simulink model "model3"  (R2023a)
settings: Solver=ode4  StartTime=0.0  StopTime=1000  FixedStep=simulation_dt  RelTol=1e-3
undefined symbols (not defined in the file or in its folder): input, k_harmonics, magnitude, simulation_dt
libraries: simulink x2
settings Model: Creator=dionl  LastModifiedBy=dionl

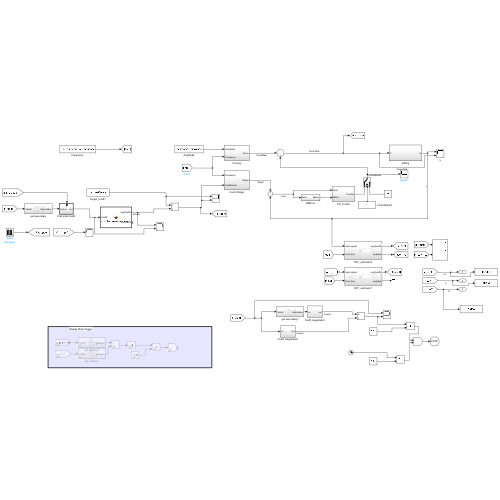
[thumbnail: Simulink's stored preview of the top-level diagram]
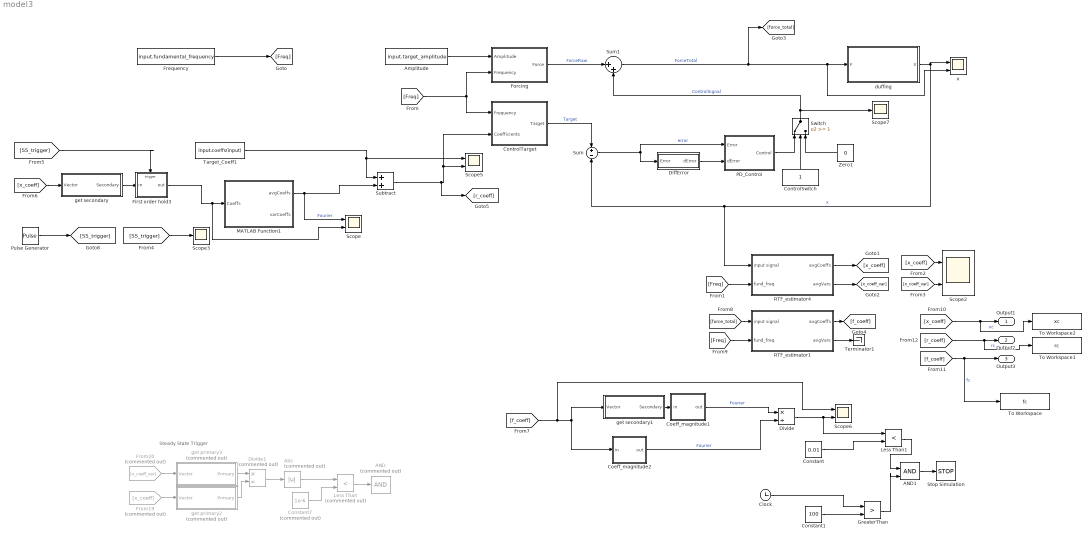
== system model3 ==
  note: Steady State Trigger
  AND : Logic  Commented=on  Inputs=1  IconShape=distinctive  AllPortsSameDT=off  OutDataTypeStr=boolean
  AND1 : Logic  IconShape=distinctive  AllPortsSameDT=off  OutDataTypeStr=boolean
  Abs : Abs  Commented=on  SaturateOnIntegerOverflow=off
  Amplitude : Constant  Value=input.target_amplitude
  Clock : Clock
  Coeff_magnitude1 : Subsystem
  Coeff_magnitude2 : Subsystem
  Constant : Constant  Value=0.01
  Constant1 : Constant  Value=100
  Constant7 : Constant  Commented=on  Value=1e-6
  ControlSwitch : Constant
  ControlTarget : Subsystem
  DiffError : Subsystem
  Divide : Product  Inputs=*/
  Divide1 : Product  Commented=on  Inputs=*/
  First order hold3 : Subsystem  TreatAsAtomicUnit=on
  Forcing : Subsystem
  Frequency : Constant  Value=input.fundamental_frequency
  From19 : From  Commented=on  GotoTag=x_coeff
  From20 : From  Commented=on  GotoTag=x_coeff_var
  GreaterThan : RelationalOperator  Operator=>  OutDataTypeStr=boolean  RndMeth=Simplest  InputSameDT=off
  Less Than : RelationalOperator  Commented=on  Operator=<  OutDataTypeStr=boolean  RndMeth=Simplest  InputSameDT=off
  Less Than1 : RelationalOperator  Operator=<  OutDataTypeStr=boolean  RndMeth=Simplest  InputSameDT=off
  MATLAB Function1 : MATLAB Function  TreatAsAtomicUnit=on
  PD_Control : Subsystem
  Pulse Generator : DiscretePulseGenerator  PulseType=Time based  Period=50  PulseWidth=5  PhaseDelay=simulation_dt
  RTF_estimator1 : Subsystem
  RTF_estimator4 : Subsystem
  Scope{,2,5..6} (4 alike) : Scope  NumInputPorts=2
  Scope3 : Scope
  Scope7 : Scope
  Stop Simulation : Stop
  Subtract : Sum
  Sum : Sum  Inputs=+|-
  Sum1 : Sum  Inputs=|++
  Switch : Switch  Threshold=1  SaturateOnIntegerOverflow=off  InputSameDT=off
  Target_Coeff1 : Constant  Value=input.coeffs(input)
  Terminator1 : Terminator
  To Workspace : ToWorkspace  VariableName=fc  SaveFormat=Timeseries  SampleTime=-1
  To Workspace1 : ToWorkspace  VariableName=rc  SaveFormat=Timeseries  SampleTime=-1
  To Workspace2 : ToWorkspace  VariableName=xc  SaveFormat=Timeseries  SampleTime=-1
  Zero1 : Constant  Value=0
  duffing : Subsystem
  get primary2 : Subsystem  Commented=on
  get primary3 : Subsystem  Commented=on
  get secondary : Subsystem
  get secondary1 : Subsystem
  x : Scope  NumInputPorts=2
  Output1 : Outport
  Output2 : Outport  Port=2
  Output3 : Outport  Port=3
  wires:
  Subtract/1 -> [r_coeff], Scope5/2, ControlTarget/2(Coefficients)
  Switch/1 -> Sum1/2, Scope7/1  "ControlSignal"
  Zero1/1 -> Switch/3
  Sum1/1 -> [force_total], x/2, duffing/1(F)  "ForceTotal"
  PD_Control/1(Control) -> Switch/1
  duffing/1(X) -> x/1, RTF_estimator4/1(input signal), Sum/2  "x"
  DiffError/1(dError) -> PD_Control/2(dError)
  Forcing/1(Force) -> Sum1/1  "ForceRaw"
  ControlSwitch/1 -> Switch/2
  Amplitude/1 -> Forcing/1(Amplitude)
  ControlTarget/1(Target) -> Sum/1  "Target"
  Frequency/1 -> [Freq]
  Sum/1 -> PD_Control/1(Error), DiffError/1(Error)  "error"
  [Freq] -> ControlTarget/1(Frequency), Forcing/2(Frequency)
  [Freq] -> RTF_estimator4/2(fund_freq)
  get primary3/1(Primary) -> Divide1/1
  Less Than/1 -> AND/1
  get primary2/1(Primary) -> Divide1/2
  Constant7/1 -> Less Than/2
  From20/1 -> get primary3/1(Vector)
  Divide1/1 -> Abs/1
  From19/1 -> get primary2/1(Vector)
  RTF_estimator4/2(avgVars) -> [x_coeff_var]
  RTF_estimator4/1(avgCoeffs) -> [x_coeff]
  [x_coeff_var] -> Scope2/2
  [x_coeff] -> Scope2/1
  [SS_trigger] -> Scope3/1
  Abs/1 -> Less Than/1
  Target_Coeff1/1 -> Subtract/1, Scope5/1
  [x_coeff] -> get secondary/1(Vector)
  get secondary/1(Secondary) -> First order hold3/1(in)
  get secondary1/1(Secondary) -> Coeff_magnitude1/1(in)
  Coeff_magnitude1/1(out) -> Divide/1  "Fourier"
  Coeff_magnitude2/1(out) -> Divide/2  "Fourier"
  Divide/1 -> Less Than1/1, Scope6/2
  [SS_trigger] -> First order hold3/Trigger
  Pulse Generator/1 -> [SS_trigger]
  [force_total] -> RTF_estimator1/1(input signal)
  [Freq] -> RTF_estimator1/2(fund_freq)
  RTF_estimator1/1(avgCoeffs) -> [f_coeff]
  RTF_estimator1/2(avgVars) -> Terminator1/1
  [f_coeff] -> Scope6/1, Coeff_magnitude2/1(in), get secondary1/1(Vector)
  Constant/1 -> Less Than1/2
  Less Than1/1 -> AND1/1
  [x_coeff] -> To Workspace2/1, Output1/1  "xc"
  [f_coeff] -> To Workspace/1, Output3/1  "fc"
  [r_coeff] -> To Workspace1/1, Output2/1  "rc"
  First order hold3/1(out) -> Scope/2, MATLAB Function1/1(Coeffs)
  MATLAB Function1/1(avgCoeffs) -> Scope/1, Subtract/2  "Fourier"
  Clock/1 -> GreaterThan/1
  Constant1/1 -> GreaterThan/2
  AND1/1 -> Stop Simulation/1
  GreaterThan/1 -> AND1/2

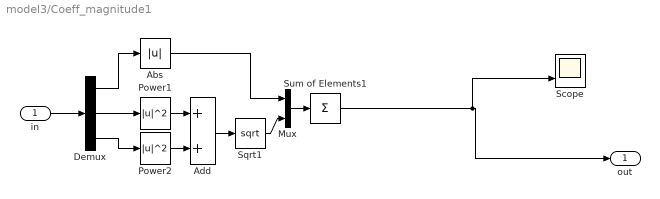
== system model3/Coeff_magnitude1 ==
  in : Inport
  Abs : Abs  SaturateOnIntegerOverflow=off
  Add : Sum
  Demux : Demux  Outputs=[1 k_harmonics k_harmonics]
  Mux : Mux  Inputs=2
  Power1 : Math  Operator=magnitude^2
  Power2 : Math  Operator=magnitude^2
  Scope : Scope  NumInputPorts=2
  Sqrt1 : Sqrt
  Sum of Elements1 : Sum  Inputs=+
  out : Outport
  wires:
  in/1 -> Demux/1
  Demux/1 -> Abs/1
  Demux/2 -> Power1/1
  Demux/3 -> Power2/1
  Power1/1 -> Add/1
  Power2/1 -> Add/2
  Add/1 -> Sqrt1/1
  Abs/1 -> Mux/1
  Sqrt1/1 -> Mux/2
  Mux/1 -> Sum of Elements1/1
  Sum of Elements1/1 -> Scope/2, out/1

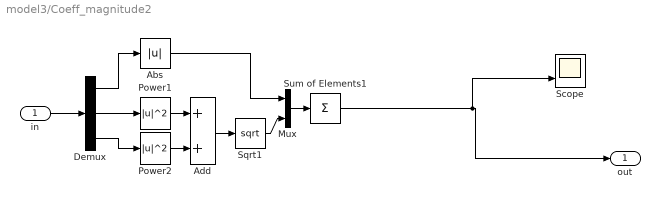
== system model3/Coeff_magnitude2 ==
  in : Inport
  Abs : Abs  SaturateOnIntegerOverflow=off
  Add : Sum
  Demux : Demux  Outputs=[1 k_harmonics k_harmonics]
  Mux : Mux  Inputs=2
  Power1 : Math  Operator=magnitude^2
  Power2 : Math  Operator=magnitude^2
  Scope : Scope  NumInputPorts=2
  Sqrt1 : Sqrt
  Sum of Elements1 : Sum  Inputs=+
  out : Outport
  wires:
  Sum of Elements1/1 -> out/1, Scope/2
  Mux/1 -> Sum of Elements1/1
  Sqrt1/1 -> Mux/2
  Abs/1 -> Mux/1
  Add/1 -> Sqrt1/1
  Power2/1 -> Add/2
  Power1/1 -> Add/1
  Demux/3 -> Power2/1
  Demux/2 -> Power1/1
  Demux/1 -> Abs/1
  in/1 -> Demux/1

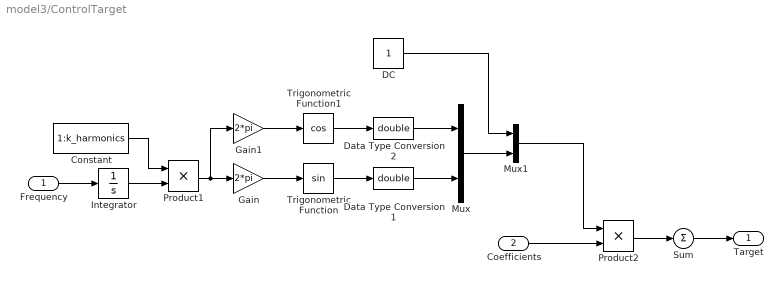
== system model3/ControlTarget ==
  Frequency : Inport
  Coefficients : Inport  Port=2
  Constant : Constant  Value=1:k_harmonics
  DC : Constant
  Data Type Conversion1 : DataTypeConversion  OutDataTypeStr=double  SaturateOnIntegerOverflow=off  RndMeth=Floor
  Data Type Conversion2 : DataTypeConversion  OutDataTypeStr=double  SaturateOnIntegerOverflow=off  RndMeth=Floor
  Gain : Gain  Gain=2*pi
  Gain1 : Gain  Gain=2*pi
  Integrator : Integrator
  Mux : Mux  Inputs=2
  Mux1 : Mux  Inputs=2
  Product1 : Product
  Product2 : Product  RndMeth=Zero
  Sum : Sum  Inputs=|+|
  Trigonometric Function : Trigonometry
  Trigonometric Function1 : Trigonometry  Operator=cos
  Target : Outport
  wires:
  Gain/1 -> Trigonometric Function/1
  Product2/1 -> Sum/1
  Gain1/1 -> Trigonometric Function1/1
  Sum/1 -> Target/1
  Frequency/1 -> Integrator/1
  Integrator/1 -> Product1/2
  Constant/1 -> Product1/1
  Trigonometric Function/1 -> Data Type Conversion1/1
  Mux1/1 -> Product2/1
  Trigonometric Function1/1 -> Data Type Conversion2/1
  Product1/1 -> Gain1/1, Gain/1
  Coefficients/1 -> Product2/2
  Data Type Conversion2/1 -> Mux/1
  Data Type Conversion1/1 -> Mux/2
  Mux/1 -> Mux1/2
  DC/1 -> Mux1/1

== system model3/DiffError ==
  Error : Inport
  Sum4 : Sum  Inputs=|-+
  Unit Delay : UnitDelay  SampleTime=-1  HasFrameUpgradeWarning=on
  Weighted Sample Time : SampleTimeMath  TsampMathOp=/
  dError : Outport
  wires:
  Unit Delay/1 -> Sum4/1
  Sum4/1 -> Weighted Sample Time/1
  Weighted Sample Time/1 -> dError/1
  Error/1 -> Unit Delay/1, Sum4/2

== system model3/First order hold3 ==
  in : Inport  LatchByDelayingOutsideSignal=on
  Trigger : TriggerPort  VariantControl=(inherit)
  out : Outport  InitialOutput=0
  wires:
  in/1 -> out/1

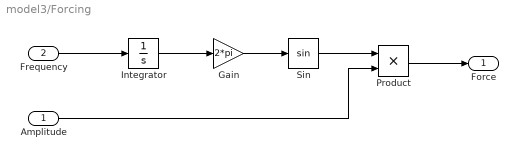
== system model3/Forcing ==
  Amplitude : Inport
  Frequency : Inport  Port=2
  Gain : Gain  Gain=2*pi
  Integrator : Integrator
  Product : Product
  Sin : Trigonometry
  Force : Outport
  wires:
  Frequency/1 -> Integrator/1
  Gain/1 -> Sin/1
  Amplitude/1 -> Product/2
  Integrator/1 -> Gain/1
  Sin/1 -> Product/1
  Product/1 -> Force/1

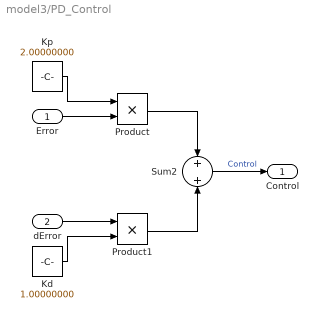
== system model3/PD_Control ==
  Error : Inport
  dError : Inport  Port=2
  Kd : Constant  Value=1.00000000
  Kp : Constant  Value=2.00000000
  Product : Product  RndMeth=Zero
  Product1 : Product  RndMeth=Zero
  Sum2 : Sum  Inputs=+|+
  Control : Outport
  wires:
  Kp/1 -> Product/1
  Kd/1 -> Product1/2
  Product/1 -> Sum2/1
  Product1/1 -> Sum2/2
  Error/1 -> Product/2
  Sum2/1 -> Control/1  "Control"
  dError/1 -> Product1/1

== system model3/RTF_estimator1 ==
  input signal : Inport
  fund_freq : Inport  Port=2
  MATLAB Function1 : MATLAB Function  TreatAsAtomicUnit=on
  Subsystem : Subsystem
  Terminator : Terminator
  avgCoeffs : Outport
  avgVars : Outport  Port=2
  wires:
  MATLAB Function1/1(avgCoeffs) -> avgCoeffs/1  "Fourier"
  MATLAB Function1/2(varCoeffs) -> avgVars/1
  Subsystem/1(Fourier1) -> MATLAB Function1/1(Coeffs)
  fund_freq/1 -> Subsystem/2(fund_freq)
  Subsystem/2(Phase1) -> Terminator/1
  input signal/1 -> Subsystem/1(input signal)

== system model3/RTF_estimator4 ==
  input signal : Inport
  fund_freq : Inport  Port=2
  MATLAB Function1 : MATLAB Function  TreatAsAtomicUnit=on
  Subsystem : Subsystem
  Terminator : Terminator
  avgCoeffs : Outport
  avgVars : Outport  Port=2
  wires:
  input signal/1 -> Subsystem/1(input signal)
  Subsystem/2(Phase1) -> Terminator/1
  fund_freq/1 -> Subsystem/2(fund_freq)
  Subsystem/1(Fourier1) -> MATLAB Function1/1(Coeffs)
  MATLAB Function1/2(varCoeffs) -> avgVars/1
  MATLAB Function1/1(avgCoeffs) -> avgCoeffs/1  "Fourier"

== system model3/duffing ==
  F : Inport
  Integrator : Integrator
  Integrator1 : Integrator
  MATLAB Function : MATLAB Function  TreatAsAtomicUnit=on
  X : Outport
  wires:
  Integrator1/1 -> MATLAB Function/2(v)
  MATLAB Function/2(dvdt) -> Integrator1/1
  MATLAB Function/1(dxdt) -> Integrator/1
  F/1 -> MATLAB Function/3(excitation)
  Integrator/1 -> MATLAB Function/1(x), X/1

== system model3/get primary2 ==
  Vector : Inport
  Demux : Demux  Outputs=[1, 1, k_harmonics-1, 1, k_harmonics-1]
  Mux : Mux  Inputs=2
  Terminator2 : Terminator
  Terminator3 : Terminator
  Terminator4 : Terminator
  Primary : Outport
  wires:
  Vector/1 -> Demux/1
  Demux/5 -> Terminator4/1
  Demux/3 -> Terminator3/1
  Mux/1 -> Primary/1
  Demux/4 -> Mux/2
  Demux/2 -> Mux/1
  Demux/1 -> Terminator2/1

== system model3/get primary3 ==
  Vector : Inport
  Demux : Demux  Outputs=[1, 1, k_harmonics-1, 1, k_harmonics-1]
  Mux : Mux  Inputs=2
  Terminator2 : Terminator
  Terminator3 : Terminator
  Terminator4 : Terminator
  Primary : Outport
  wires:
  Demux/1 -> Terminator2/1
  Demux/2 -> Mux/1
  Demux/4 -> Mux/2
  Mux/1 -> Primary/1
  Demux/3 -> Terminator3/1
  Demux/5 -> Terminator4/1
  Vector/1 -> Demux/1

== system model3/get secondary ==
  Vector : Inport
  Demux : Demux  Outputs=[1, 1, k_harmonics-1, 1, k_harmonics-1]
  Gain1 : Gain  Gain=0
  Gain2 : Gain  Gain=0
  Gain3 : Gain  Gain=0
  Mux : Mux  Inputs=5
  Secondary : Outport
  wires:
  Vector/1 -> Demux/1
  Mux/1 -> Secondary/1
  Demux/4 -> Gain1/1
  Demux/2 -> Gain3/1
  Demux/1 -> Gain2/1
  Gain2/1 -> Mux/1
  Demux/3 -> Mux/3
  Demux/5 -> Mux/5
  Gain3/1 -> Mux/2
  Gain1/1 -> Mux/4

== system model3/get secondary1 ==
  Vector : Inport
  Demux : Demux  Outputs=[1, 1, k_harmonics-1, 1, k_harmonics-1]
  Gain1 : Gain  Gain=0
  Gain2 : Gain  Gain=0
  Gain3 : Gain  Gain=0
  Mux : Mux  Inputs=5
  Secondary : Outport
  wires:
  Gain1/1 -> Mux/4
  Gain3/1 -> Mux/2
  Demux/5 -> Mux/5
  Demux/3 -> Mux/3
  Gain2/1 -> Mux/1
  Demux/1 -> Gain2/1
  Demux/2 -> Gain3/1
  Demux/4 -> Gain1/1
  Mux/1 -> Secondary/1
  Vector/1 -> Demux/1

== system model3/RTF_estimator1/Subsystem ==
  input signal : Inport
  fund_freq : Inport  Port=2
  Fourier Series 2 : Subsystem
  Harmonic Basis Gen1 : Subsystem
  Fourier1 : Outport
  Phase1 : Outport  Port=2
  wires:
  Harmonic Basis Gen1/1(harmonic_basis) -> Fourier Series 2/2(harmonic basis)
  fund_freq/1 -> Fourier Series 2/3(fundamental frequency), Harmonic Basis Gen1/1(fund_freq)
  Fourier Series 2/1(Fourier) -> Fourier1/1
  input signal/1 -> Fourier Series 2/1(input signal)
  Fourier Series 2/2(Phase) -> Phase1/1

== system model3/RTF_estimator4/Subsystem ==
  input signal : Inport
  fund_freq : Inport  Port=2
  Fourier Series 2 : Subsystem
  Harmonic Basis Gen1 : Subsystem
  Fourier1 : Outport
  Phase1 : Outport  Port=2
  wires:
  Fourier Series 2/2(Phase) -> Phase1/1
  input signal/1 -> Fourier Series 2/1(input signal)
  Fourier Series 2/1(Fourier) -> Fourier1/1
  fund_freq/1 -> Harmonic Basis Gen1/1(fund_freq), Fourier Series 2/3(fundamental frequency)
  Harmonic Basis Gen1/1(harmonic_basis) -> Fourier Series 2/2(harmonic basis)

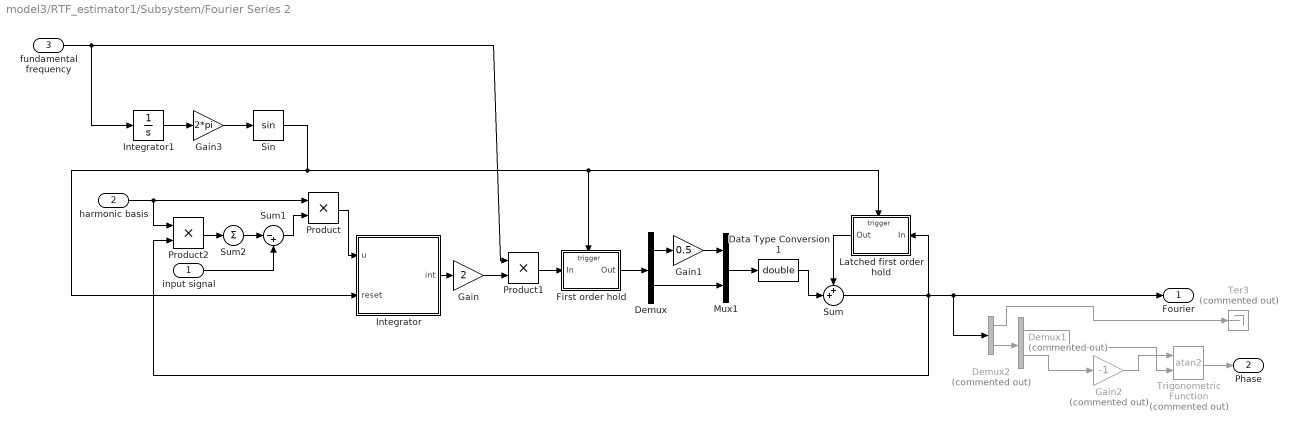
== system model3/RTF_estimator1/Subsystem/Fourier Series 2 ==
  input signal : Inport
  harmonic basis : Inport  Port=2
  fundamental frequency : Inport  Port=3
  Data Type Conversion1 : DataTypeConversion  OutDataTypeStr=double  SaturateOnIntegerOverflow=off  RndMeth=Floor
  Demux : Demux  Outputs=[1 -1]
  Demux1 : Demux  Commented=on  Outputs=2
  Demux2 : Demux  Commented=on  Outputs=[1 -1]
  First order hold : Subsystem  TreatAsAtomicUnit=on
  Gain : Gain  Gain=2
  Gain1 : Gain  Gain=0.5
  Gain2 : Gain  Commented=on  Gain=-1
  Gain3 : Gain  Gain=2*pi
  Integrator : Subsystem
  Integrator1 : Integrator
  Latched first order hold : Subsystem  TreatAsAtomicUnit=on
  Mux1 : Mux  Inputs=2
  Product : Product  RndMeth=Zero
  Product1 : Product  RndMeth=Zero
  Product2 : Product  RndMeth=Zero
  Sin : Trigonometry
  Sum : Sum  Tag=Test  Inputs=++|
  Sum1 : Sum  Inputs=|-+
  Sum2 : Sum  Inputs=|+|
  Ter3 : Terminator  Commented=on
  Trigonometric Function : Trigonometry  Commented=on  Operator=atan2
  Fourier : Outport
  Phase : Outport  Port=2
  wires:
  Product1/1 -> First order hold/1(In)
  Gain/1 -> Product1/2
  Sin/1 -> Integrator/2(reset), First order hold/Trigger, Latched first order hold/Trigger
  Integrator/1(int) -> Gain/1
  Demux/1 -> Gain1/1
  Gain1/1 -> Mux1/1
  Demux/2 -> Mux1/2
  First order hold/1(Out) -> Demux/1
  Mux1/1 -> Data Type Conversion1/1
  Data Type Conversion1/1 -> Sum/2
  Sum/1 -> Product2/2, Latched first order hold/1(In), Fourier/1, Demux2/1
  Latched first order hold/1(Out) -> Sum/1
  Sum1/1 -> Product/2
  Product2/1 -> Sum2/1
  input signal/1 -> Sum1/2
  harmonic basis/1 -> Product/1, Product2/1
  Sum2/1 -> Sum1/1
  Trigonometric Function/1 -> Phase/1
  Product/1 -> Integrator/1(u)
  Demux1/1 -> Trigonometric Function/2
  Demux1/2 -> Gain2/1
  Gain2/1 -> Trigonometric Function/1
  Demux2/2 -> Demux1/1
  Demux2/1 -> Ter3/1
  Gain3/1 -> Sin/1
  Integrator1/1 -> Gain3/1
  fundamental frequency/1 -> Integrator1/1, Product1/1

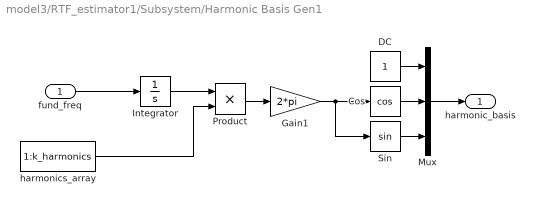
== system model3/RTF_estimator1/Subsystem/Harmonic Basis Gen1 ==
  fund_freq : Inport
  Cos : Trigonometry  Operator=cos
  DC : Constant
  Gain1 : Gain  Gain=2*pi
  Integrator : Integrator
  Mux : Mux  Inputs=3
  Product : Product
  Sin : Trigonometry
  harmonics_array : Constant  Value=1:k_harmonics
  harmonic_basis : Outport  OutDataTypeStr=double  SampleTime=0
  wires:
  DC/1 -> Mux/1
  fund_freq/1 -> Integrator/1
  harmonics_array/1 -> Product/2
  Sin/1 -> Mux/3
  Product/1 -> Gain1/1
  Cos/1 -> Mux/2
  Integrator/1 -> Product/1
  Mux/1 -> harmonic_basis/1
  Gain1/1 -> Cos/1, Sin/1

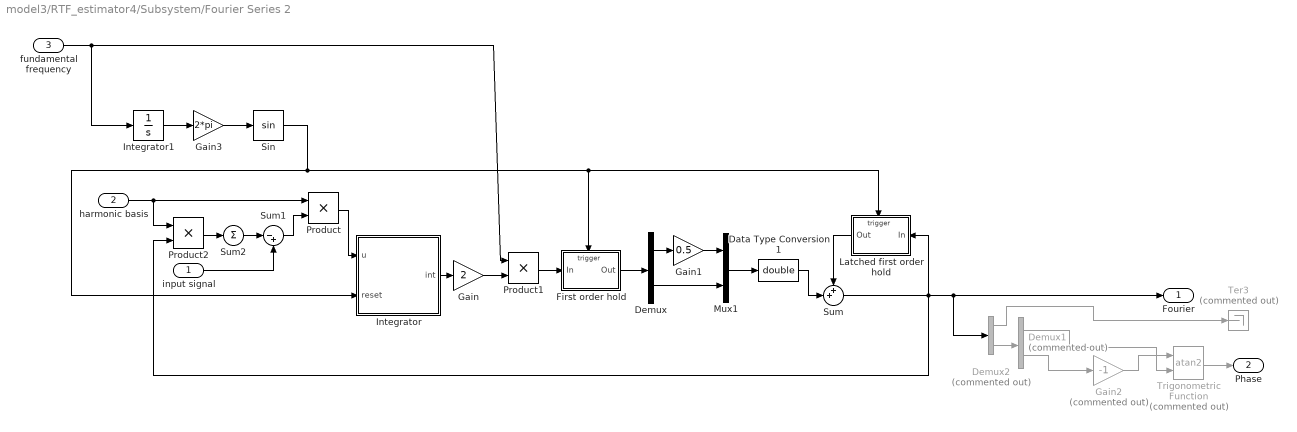
== system model3/RTF_estimator4/Subsystem/Fourier Series 2 ==
  input signal : Inport
  harmonic basis : Inport  Port=2
  fundamental frequency : Inport  Port=3
  Data Type Conversion1 : DataTypeConversion  OutDataTypeStr=double  SaturateOnIntegerOverflow=off  RndMeth=Floor
  Demux : Demux  Outputs=[1 -1]
  Demux1 : Demux  Commented=on  Outputs=2
  Demux2 : Demux  Commented=on  Outputs=[1 -1]
  First order hold : Subsystem  TreatAsAtomicUnit=on
  Gain : Gain  Gain=2
  Gain1 : Gain  Gain=0.5
  Gain2 : Gain  Commented=on  Gain=-1
  Gain3 : Gain  Gain=2*pi
  Integrator : Subsystem
  Integrator1 : Integrator
  Latched first order hold : Subsystem  TreatAsAtomicUnit=on
  Mux1 : Mux  Inputs=2
  Product : Product  RndMeth=Zero
  Product1 : Product  RndMeth=Zero
  Product2 : Product  RndMeth=Zero
  Sin : Trigonometry
  Sum : Sum  Tag=Test  Inputs=++|
  Sum1 : Sum  Inputs=|-+
  Sum2 : Sum  Inputs=|+|
  Ter3 : Terminator  Commented=on
  Trigonometric Function : Trigonometry  Commented=on  Operator=atan2
  Fourier : Outport
  Phase : Outport  Port=2
  wires:
  fundamental frequency/1 -> Product1/1, Integrator1/1
  Integrator1/1 -> Gain3/1
  Gain3/1 -> Sin/1
  Demux2/1 -> Ter3/1
  Demux2/2 -> Demux1/1
  Gain2/1 -> Trigonometric Function/1
  Demux1/2 -> Gain2/1
  Demux1/1 -> Trigonometric Function/2
  Product/1 -> Integrator/1(u)
  Trigonometric Function/1 -> Phase/1
  Sum2/1 -> Sum1/1
  harmonic basis/1 -> Product2/1, Product/1
  input signal/1 -> Sum1/2
  Product2/1 -> Sum2/1
  Sum1/1 -> Product/2
  Latched first order hold/1(Out) -> Sum/1
  Sum/1 -> Demux2/1, Fourier/1, Latched first order hold/1(In), Product2/2
  Data Type Conversion1/1 -> Sum/2
  Mux1/1 -> Data Type Conversion1/1
  First order hold/1(Out) -> Demux/1
  Demux/2 -> Mux1/2
  Gain1/1 -> Mux1/1
  Demux/1 -> Gain1/1
  Integrator/1(int) -> Gain/1
  Sin/1 -> Latched first order hold/Trigger, First order hold/Trigger, Integrator/2(reset)
  Gain/1 -> Product1/2
  Product1/1 -> First order hold/1(In)

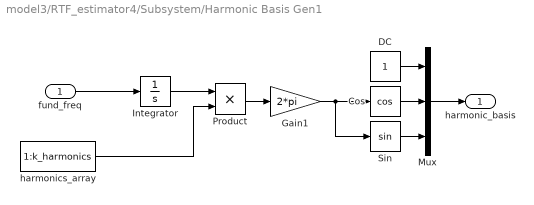
== system model3/RTF_estimator4/Subsystem/Harmonic Basis Gen1 ==
  fund_freq : Inport
  Cos : Trigonometry  Operator=cos
  DC : Constant
  Gain1 : Gain  Gain=2*pi
  Integrator : Integrator
  Mux : Mux  Inputs=3
  Product : Product
  Sin : Trigonometry
  harmonics_array : Constant  Value=1:k_harmonics
  harmonic_basis : Outport  OutDataTypeStr=double  SampleTime=0
  wires:
  Gain1/1 -> Sin/1, Cos/1
  Mux/1 -> harmonic_basis/1
  Integrator/1 -> Product/1
  Cos/1 -> Mux/2
  Product/1 -> Gain1/1
  Sin/1 -> Mux/3
  harmonics_array/1 -> Product/2
  fund_freq/1 -> Integrator/1
  DC/1 -> Mux/1

== system model3/RTF_estimator1/Subsystem/Fourier Series 2/First order hold ==
  In : Inport  LatchByDelayingOutsideSignal=on
  Trigger : TriggerPort  VariantControl=(inherit)
  Out : Outport
  wires:
  In/1 -> Out/1

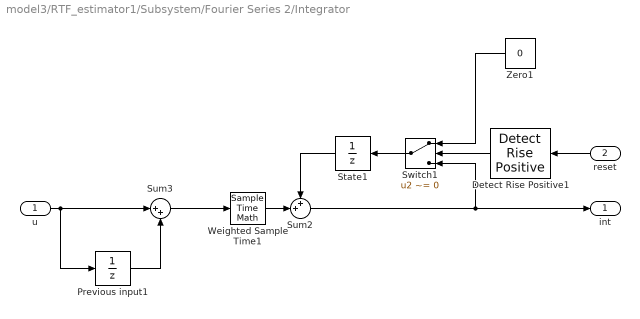
== system model3/RTF_estimator1/Subsystem/Fourier Series 2/Integrator ==
  u : Inport
  reset : Inport  Port=2
  Detect Rise Positive1 : simulink/Logic and Bit Operations/Detect Rise Positive  vinit=0  OutDataTypeStr=uint8
  Previous input1 : UnitDelay  SampleTime=-1  HasFrameUpgradeWarning=on
  State1 : UnitDelay  SampleTime=-1  HasFrameUpgradeWarning=on
  Sum2 : Sum  Inputs=++|
  Sum3 : Sum  Inputs=|++
  Switch1 : Switch  Criteria=u2 ~= 0  SaturateOnIntegerOverflow=off  InputSameDT=off
  Weighted Sample Time1 : SampleTimeMath  TsampMathOp=*  weightValue=0.5
  Zero1 : Constant  Value=0
  int : Outport
  wires:
  Detect Rise Positive1/1 -> Switch1/2
  Zero1/1 -> Switch1/1
  Switch1/1 -> State1/1
  reset/1 -> Detect Rise Positive1/1
  Previous input1/1 -> Sum3/2
  u/1 -> Previous input1/1, Sum3/1
  Sum3/1 -> Weighted Sample Time1/1
  Weighted Sample Time1/1 -> Sum2/2
  Sum2/1 -> int/1, Switch1/3
  State1/1 -> Sum2/1

== system model3/RTF_estimator1/Subsystem/Fourier Series 2/Latched first order hold ==
  In : Inport  LatchByDelayingOutsideSignal=on
  Trigger : TriggerPort  VariantControl=(inherit)
  Out : Outport
  wires:
  In/1 -> Out/1

== system model3/RTF_estimator4/Subsystem/Fourier Series 2/First order hold ==
  In : Inport  LatchByDelayingOutsideSignal=on
  Trigger : TriggerPort  VariantControl=(inherit)
  Out : Outport
  wires:
  In/1 -> Out/1

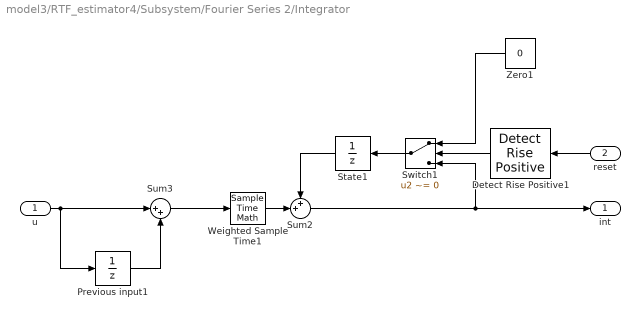
== system model3/RTF_estimator4/Subsystem/Fourier Series 2/Integrator ==
  u : Inport
  reset : Inport  Port=2
  Detect Rise Positive1 : simulink/Logic and Bit Operations/Detect Rise Positive  vinit=0  OutDataTypeStr=uint8
  Previous input1 : UnitDelay  SampleTime=-1  HasFrameUpgradeWarning=on
  State1 : UnitDelay  SampleTime=-1  HasFrameUpgradeWarning=on
  Sum2 : Sum  Inputs=++|
  Sum3 : Sum  Inputs=|++
  Switch1 : Switch  Criteria=u2 ~= 0  SaturateOnIntegerOverflow=off  InputSameDT=off
  Weighted Sample Time1 : SampleTimeMath  TsampMathOp=*  weightValue=0.5
  Zero1 : Constant  Value=0
  int : Outport
  wires:
  State1/1 -> Sum2/1
  Sum2/1 -> Switch1/3, int/1
  Weighted Sample Time1/1 -> Sum2/2
  Sum3/1 -> Weighted Sample Time1/1
  u/1 -> Sum3/1, Previous input1/1
  Previous input1/1 -> Sum3/2
  reset/1 -> Detect Rise Positive1/1
  Switch1/1 -> State1/1
  Zero1/1 -> Switch1/1
  Detect Rise Positive1/1 -> Switch1/2

== system model3/RTF_estimator4/Subsystem/Fourier Series 2/Latched first order hold ==
  In : Inport  LatchByDelayingOutsideSignal=on
  Trigger : TriggerPort  VariantControl=(inherit)
  Out : Outport
  wires:
  In/1 -> Out/1

== matlab function model3/RTF_estimator1/MATLAB Function1 ==
  data: Coeffs input; avgCoeffs output; varCoeffs output
function [avgCoeffs, varCoeffs] = exponentialAverageWithVariance(Coeffs)
% Exponential Moving Average (EMA) and Variance (EMV) for Fourier Coefficients

% Tuning parameter
alpha = 5e-4;  % 0.001 (slow, smooth) to 0.1 (fast, responsive)

% Persistent storage
persistent avg sqAvg
if isempty(avg)
    avg = Coeffs;
    sqAvg = Coeffs.^2;
end

% EMA update
avg = alpha * Coeffs + (1 - alpha) * avg;

% EMA of square
sqAvg = alpha * (Coeffs.^2) + (1 - alpha) * sqAvg;

% Variance = E[x^2] - (E[x])^2
varCoeffs = sqAvg - avg.^2;

% Output
avgCoeffs = avg;
end

== matlab function model3/duffing/MATLAB Function ==
  data: x input; dxdt output; v input; excitation input; dvdt output
function [dxdt, dvdt] = duffingDerivatives(x, v, excitation)
% Duffing oscillator derivatives
%
% Inputs:
%   x - displacement
%   v - velocity
%   excitation - external excitation signal
%
% Outputs:
%   dx/dt dv/dt

% Define Duffing parameters

% stable duffing
delta = 0.2;    % damping
alpha = +1;     % linear stiffness
beta  = 1;      % nonlinear stiffness

% bi-stable duffing
% delta = 0.2;    % damping
% alpha = -1;     % linear stiffness
% beta  = 1;      % nonlinear stiffness

% bi-stable duffing from Rezaee, Renson: https://doi.org/10.1137/23M1587774
% delta = 0.1;    % damping
% alpha = -4;     % linear stiffness
% beta  = 2;      % nonlinear stiffness


% Duffing equation derivatives
dxdt = v;
dvdt = excitation - delta*v - alpha*x - beta*x^3;

end

== matlab function model3/MATLAB Function1 ==
  data: Coeffs input; avgCoeffs output; varCoeffs output
function [avgCoeffs, varCoeffs] = exponentialAverageWithVariance(Coeffs)
% Exponential Moving Average (EMA) and Variance (EMV) for Fourier Coefficients

% Tuning parameter
alpha = 5e-4;  % 0.001 (slow, smooth) to 0.1 (fast, responsive)

% Persistent storage
persistent avg sqAvg
if isempty(avg)
    avg = Coeffs;
    sqAvg = Coeffs.^2;
end

% EMA update
avg = alpha * Coeffs + (1 - alpha) * avg;

% EMA of square
sqAvg = alpha * (Coeffs.^2) + (1 - alpha) * sqAvg;

% Variance = E[x^2] - (E[x])^2
varCoeffs = sqAvg - avg.^2;

% Output
avgCoeffs = avg;
end

== matlab function model3/RTF_estimator4/MATLAB Function1 ==
  data: Coeffs input; avgCoeffs output; varCoeffs output
function [avgCoeffs, varCoeffs] = exponentialAverageWithVariance(Coeffs)
% Exponential Moving Average (EMA) and Variance (EMV) for Fourier Coefficients

% Tuning parameter
alpha = 5e-4;  % 0.001 (slow, smooth) to 0.1 (fast, responsive)

% Persistent storage
persistent avg sqAvg
if isempty(avg)
    avg = Coeffs;
    sqAvg = Coeffs.^2;
end

% EMA update
avg = alpha * Coeffs + (1 - alpha) * avg;

% EMA of square
sqAvg = alpha * (Coeffs.^2) + (1 - alpha) * sqAvg;

% Variance = E[x^2] - (E[x])^2
varCoeffs = sqAvg - avg.^2;

% Output
avgCoeffs = avg;
end
